simulink model "designation_loop"  (R2025b)
settings: Solver=ode45  StartTime=0.0  StopTime=0.45  RelTol=1e-3
values from neighbouring files (symbols this model uses):
  dz = 0*(pi/180)    (= 0)    [designation_loop_design.m]
  Kd = 2.695    [Margin.m]    (also in designation_loop_design.m = 2.69488642049)
  Kp = 72.95    [Margin.m]    (also in designation_loop_design.m = 72.951065746)
  w_sat = 1400*(pi/180)    (= 24.4346095279)    [designation_loop_design.m]
settings Model: Creator=ADMIN  LastModifiedBy=ADMIN

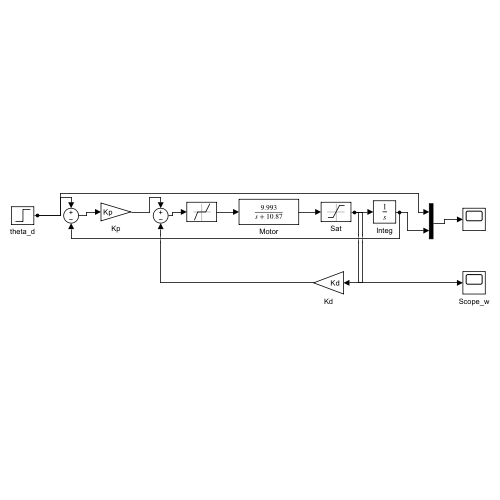
[thumbnail: Simulink's stored preview of the top-level diagram]
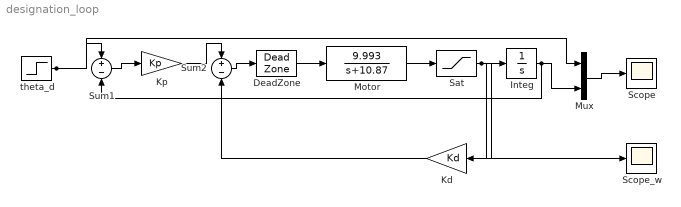
== system designation_loop ==
  DeadZone : DeadZone  LowerValue=-dz  UpperValue=dz
  Integ : Integrator
  Kd : Gain  Gain=Kd
  Kp : Gain  Gain=Kp
  Motor : TransferFcn  Numerator=[9.993]  Denominator=[1 10.87]
  Mux : Mux  Inputs=2
  Sat : Saturate  UpperLimit=w_sat  LowerLimit=-w_sat
  Scope : Scope
  Scope_w : Scope
  Sum1 : Sum  Inputs=+-
  Sum2 : Sum  Inputs=+-
  theta_d : Step  Time=0  SampleTime=0
  wires:
  theta_d/1 -> Sum1/1, Mux/1
  Sum1/1 -> Kp/1
  Kp/1 -> Sum2/1
  Sum2/1 -> DeadZone/1
  DeadZone/1 -> Motor/1
  Motor/1 -> Sat/1
  Sat/1 -> Integ/1, Kd/1, Scope_w/1
  Kd/1 -> Sum2/2
  Integ/1 -> Sum1/2, Mux/2
  Mux/1 -> Scope/1
